simulink model "untitled"  (R2016a)
settings: Solver=VariableStepAuto  StartTime=0.0  StopTime=50  RelTol=1e-3
settings Model: Creator=Student  LastModifiedBy=Student

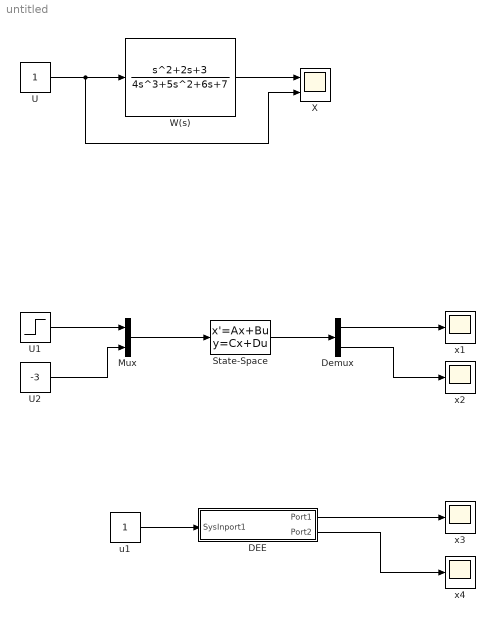
== system untitled ==
  DEE : Subsystem  mask(Differential Equation Editor (DEE)){}
      settings: OpenFcn=diffeqed
      mask Display: disp('Differential Equation\n Editor')
  Demux : Demux  Outputs=2
  Mux : Mux  Inputs=2
  State-Space : StateSpace  A=[-1 -1;1 0]  B=[1 0;0 1]  C=[1 0;0 1]  D=[0 0;0 0]  X0=[0 0]
  U : Constant
  U1 : Step  SampleTime=0
  U2 : Constant  Value=-3
  W(s) : TransferFcn  Numerator=[1 2 3]  Denominator=[4 5 6 7]
  X : Scope  NumInputPorts=2
  u1 : Constant
  x{1..4} (4 alike) : Scope
  wires:
  U/1 -> X/2, W(s)/1
  W(s)/1 -> X/1
  U1/1 -> Mux/1
  U2/1 -> Mux/2
  Mux/1 -> State-Space/1
  State-Space/1 -> Demux/1
  Demux/1 -> x1/1
  Demux/2 -> x2/1
  u1/1 -> DEE/1(SysInport1)
  DEE/1(Port1) -> x3/1
  DEE/2(Port2) -> x4/1

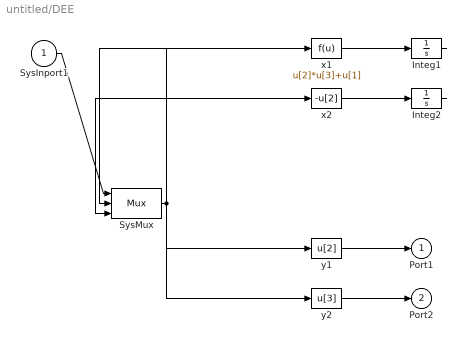
== system untitled/DEE ==
  SysInport1 : Inport
  Integ1 : Integrator
  Integ2 : Integrator
  SysMux : Mux  Inputs=3
  x1 : Fcn  Expr=u[2]*u[3]+u[1]
  x2 : Fcn  Expr=-u[2]
  y1 : Fcn  Expr=u[2]
  y2 : Fcn  Expr=u[3]
  Port1 : Outport
  Port2 : Outport  Port=2
  wires:
  SysInport1/1 -> SysMux/1
  SysMux/1 -> x1/1, x2/1, y1/1, y2/1
  x1/1 -> Integ1/1
  Integ1/1 -> SysMux/2
  x2/1 -> Integ2/1
  Integ2/1 -> SysMux/3
  y1/1 -> Port1/1
  y2/1 -> Port2/1
